simulink model "Logical_Ventilation"  (R2025b)
settings: Solver=VariableStepAuto  StartTime=0.0  StopTime=inf  RelTol=1e-3
PostLoadFcn:
  | load rel_humidity.mat;
  | load rel_humidity_heatedwire.mat;
  | load rel_humidityInput.mat;
libraries: slident x2, SignalEditorBlockLib x1
(part 3 of 3)

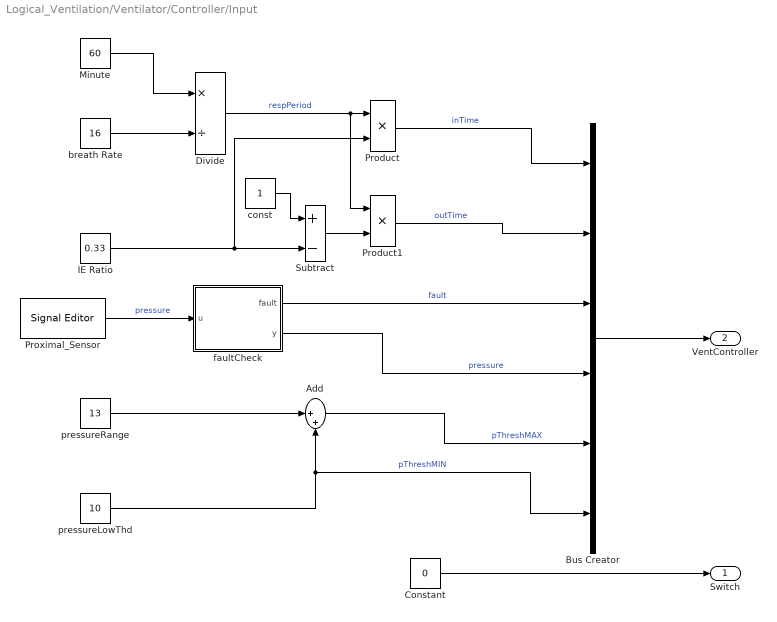
== system Logical_Ventilation/Ventilator/Controller/Input ==
  Add : Sum  Inputs=|++
  Bus Creator : BusCreator  Inputs=6
  Constant : Constant  Value=0
  Divide : Product  Inputs=*/
  IE Ratio : Constant  Value=0.33
  Minute : Constant  Value=60
  Product : Product
  Product1 : Product
  Proximal_Sensor : SignalEditorBlockLib/Signal Editor  FileName=pressure.mat  ActiveScenario=Scenario  ActiveSignal=Signal 1  IsBus=off  OutputBusObjectStr=Bus: BusObject  SampleTime=0  Interpolate=off  ZeroCross=off  OutputAfterFinalValue=Setting to zero  Unit=inherit  PreserveSignalName=on  ApplySigPropsToAllScenarios=on  ApplySigPropsToAllSignals=off  SignalPropertySource=Dialog parameters
  Subtract : Sum  Inputs=+-
  breath Rate : Constant  Value=16
  const : Constant
  faultCheck : MATLAB Function  TreatAsAtomicUnit=on
  pressureLowThd : Constant  Value=10
  pressureRange : Constant  Value=13
  Switch : Outport
  VentController : Outport  Port=2  OutDataTypeStr=Bus: VentController
  wires:
  pressureLowThd/1 -> Add/2, Bus Creator/6  "pThreshMIN"
  faultCheck/2(y) -> Bus Creator/4  "pressure"
  Product/1 -> Bus Creator/1  "inTime"
  faultCheck/1(fault) -> Bus Creator/3  "fault"
  IE Ratio/1 -> Subtract/2, Product/2
  Subtract/1 -> Product1/2
  Proximal_Sensor/1 -> faultCheck/1(u)  "pressure"
  Constant/1 -> Switch/1
  breath Rate/1 -> Divide/2
  const/1 -> Subtract/1
  pressureRange/1 -> Add/1
  Minute/1 -> Divide/1
  Add/1 -> Bus Creator/5  "pThreshMAX"
  Product1/1 -> Bus Creator/2  "outTime"
  Divide/1 -> Product1/1, Product/1  "respPeriod"
  Bus Creator/1 -> VentController/1

== system Logical_Ventilation/Ventilator/Expiratory_System/Expiratory_Tube ==
  Bus Element In1 : Inport  PortName=ExpirTube_Temp
  CheckValve : Subsystem
      settings: PortSchema="{\"entries\":[{\"content\":{\"headerSize\":26,\"margin\":15,\"minimumSpacing\":25,\"sides\":[{\"content\":{},\"type\":\"ConnectorPlacement.EquallySpacedRectSide\",\"uuid\":\"30d5a539-2c7a-40a6-b159-872080309fb0\"},{\"content\":{\"side\":\"RIGHT\"},\"type\":\"ConnectorPlacement.EquallySpacedRectSide\",\"uuid\":\"9c23b845-c6d3-461f-9717-3c81fce4740e\"},{\"content\":{\"side\":\"TOP\"},\"type\":\"ConnectorPlacement.EquallySpacedRectSide\",\"uuid\":\"23e2f61e-2083-47d3-9d3a-aca5cd4f1fc6\"}]},\"type\":\"ConnectorPlacement.EquallySpacedConnector\",\"uuid\":\"a2e9d942-417e-49d1-8834-66036fdf29fe\"}],\"packageUris\":[\"http://schema.mathworks.com/mf0/Connector/R2020b\"],\"version\":\"1.0\"}"
  Temp_RH_Sensor : Subsystem
      settings: PortSchema="{\"entries\":[{\"content\":{\"headerSize\":26,\"margin\":15,\"minimumSpacing\":25,\"sides\":[{\"content\":{},\"type\":\"ConnectorPlacement.EquallySpacedRectSide\",\"uuid\":\"30d5a539-2c7a-40a6-b159-872080309fb0\"},{\"content\":{\"connectorIds\":[\"In1\"],\"side\":\"RIGHT\"},\"type\":\"ConnectorPlacement.EquallySpacedRectSide\",\"uuid\":\"9c23b845-c6d3-461f-9717-3c81fce4740e\"},{\"content\":{\"side\":\"TOP\"},\"type\":\"ConnectorPlacement.EquallySpacedRectSide\",\"uuid\":\"23e2f61e-2083-47d3-9d3a-aca5cd4f1fc6\"}]},\"type\":\"ConnectorPlacement.EquallySpacedConnector\",\"uuid\":\"a2e9d942-417e-49d1-8834-66036fdf29fe\"}],\"packageUris\":[\"http://schema.mathworks.com/mf0/Connector/R2020b\"],\"version\":\"1.0\"}"
  wires:
  Bus Element In1/1 -> Temp_RH_Sensor/1(ExpSens_T)

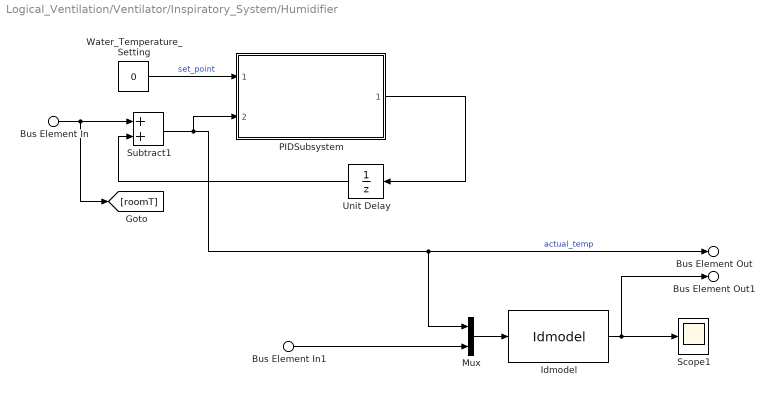
== system Logical_Ventilation/Ventilator/Inspiratory_System/Humidifier ==
  Bus Element In : Inport  PortName=InValveT  Element=Room_T
  Bus Element In1 : Inport  Port=2  PortName=InValveH  Element=Room_H
  Idmodel : slident/Models/Idmodel  sys=mp  IC=0  noi=on  seed=[]
  Mux : Mux  Inputs=2
  PIDSubsystem : Subsystem  ClipboardFcn=|  SystemSampleTime=0.05  ReferencedSubsystem=PIDSubsystem
      | Ts = 0.05;
      | Kp = 0.1;
      | Ki = 0.5;
      settings: PermitHierarchicalResolution=None
  Scope1 : Scope
      settings: ActiveDisplayYMinimum=-0.00289  ActiveDisplayYMaximum=0.02607
  Subtract1 : Sum
  Unit Delay : UnitDelay  SampleTime=-1  HasFrameUpgradeWarning=on
  Water_Temperature_Setting : Constant  Value=0
  Bus Element Out : Outport  PortName=HumidT  Element=Water_T
  Bus Element Out1 : Outport  Port=2  PortName=HumidH  Element=Humidifier_H
  wires:
  PIDSubsystem/1 -> Unit Delay/1
  Unit Delay/1 -> Subtract1/2
  Water_Temperature_Setting/1 -> PIDSubsystem/1  "set_point"
  Bus Element In/1 -> [roomT], Subtract1/1
  Subtract1/1 -> Bus Element Out/1, Mux/1, PIDSubsystem/2  "actual_temp"
  Bus Element In1/1 -> Mux/2
  Idmodel/1 -> Bus Element Out1/1, Scope1/1
  Mux/1 -> Idmodel/1

== system Logical_Ventilation/Ventilator/Inspiratory_System/Inhalation_Valve ==
  Room Relative Humidity (g) : FromWorkspace  VariableName=relh_input  OutDataTypeStr=double
  Room Temp (degC) : Constant  Value=20
  Bus Element Out : Outport  PortName=InspT  Element=Room_T
  Bus Element Out1 : Outport  Port=2  PortName=InspH  Element=Room_H
  wires:
  Room Temp (degC)/1 -> Bus Element Out/1
  Room Relative Humidity (g)/1 -> Bus Element Out1/1

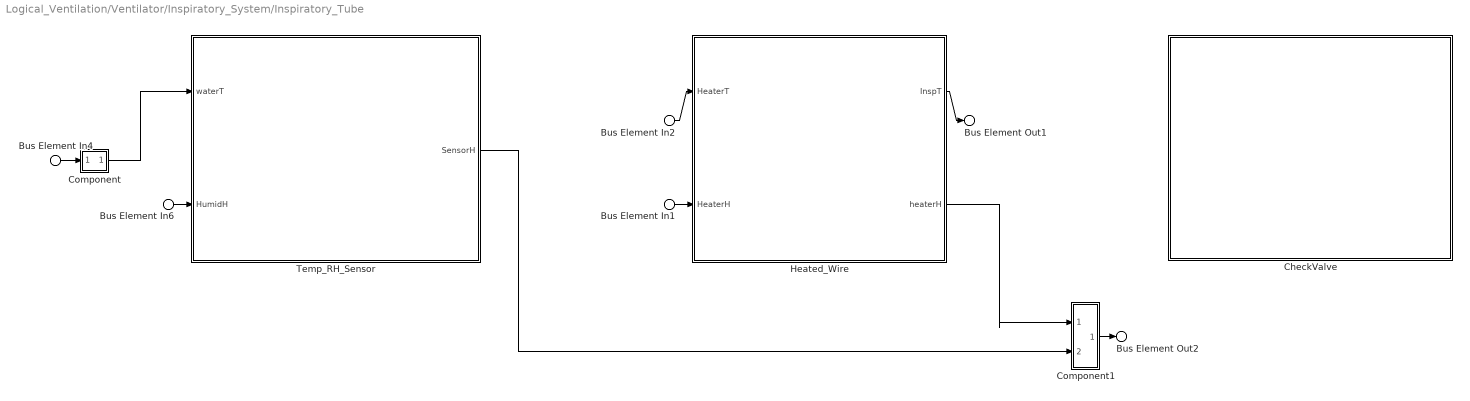
== system Logical_Ventilation/Ventilator/Inspiratory_System/Inspiratory_Tube ==
  Bus Element In1 : Inport  PortName=HumidH
  Bus Element In6 : Inport  PortName=HumidH
  Bus Element In2 : Inport  Port=2  PortName=HumidT
  Bus Element In4 : Inport  Port=2  PortName=HumidT
  CheckValve : Subsystem
      settings: PortSchema="{\"entries\":[{\"content\":{\"headerSize\":26,\"margin\":15,\"minimumSpacing\":25,\"sides\":[{\"content\":{},\"type\":\"ConnectorPlacement.EquallySpacedRectSide\",\"uuid\":\"c28154e5-eaf5-480f-8066-17b2d40a2bdd\"},{\"content\":{\"side\":\"RIGHT\"},\"type\":\"ConnectorPlacement.EquallySpacedRectSide\",\"uuid\":\"c3e70359-248e-4787-971d-b6b9bea98e42\"},{\"content\":{\"side\":\"TOP\"},\"type\":\"ConnectorPlacement.EquallySpacedRectSide\",\"uuid\":\"d2a5be48-e58c-43bd-a458-b63b8b525dc1\"}]},\"type\":\"ConnectorPlacement.EquallySpacedConnector\",\"uuid\":\"4afb880b-0c9a-4048-831b-5d1f8f54d79c\"}],\"packageUris\":[\"http://schema.mathworks.com/mf0/Connector/R2020b\"],\"version\":\"1.0\"}"
  Component : Subsystem
      settings: PortSchema="{\"entries\":[{\"content\":{\"margin\":10,\"minimumSpacing\":15,\"sides\":[{\"content\":{\"connectorIds\":[\"In1\"]},\"type\":\"ConnectorPlacement.EquallySpacedRectSide\",\"uuid\":\"ad8c2344-4809-4832-ae62-0542e39a6856\"},{\"content\":{\"connectorIds\":[\"Out1\"],\"side\":\"RIGHT\"},\"type\":\"ConnectorPlacement.EquallySpacedRectSide\",\"uuid\":\"33082802-14bb-48ab-8efd-54a486fc0ece\"},{\"content\":{\"side\":\"TOP\"},\"type\":\"ConnectorPlacement.EquallySpacedRectSide\",\"uuid\":\"4e03c195-d332-43d0-aeb9-c5e6eda740ab\"}]},\"type\":\"ConnectorPlacement.EquallySpacedConnector\",\"uuid\":\"d0446147-b41e-4bb8-8f56-ac2a90a5b24d\"}],\"packageUris\":[\"http://schema.mathworks.com/mf0/Connector/R2020b\"],\"version\":\"1.0\"}"
  Component1 : Subsystem
      settings: PortSchema="{\"entries\":[{\"content\":{\"margin\":10,\"minimumSpacing\":15,\"sides\":[{\"content\":{\"connectorIds\":[\"In1\",\"In2\"]},\"type\":\"ConnectorPlacement.EquallySpacedRectSide\",\"uuid\":\"18e365e9-4ccc-4943-ae85-7abdeaed82a1\"},{\"content\":{\"connectorIds\":[\"Out1\"],\"side\":\"RIGHT\"},\"type\":\"ConnectorPlacement.EquallySpacedRectSide\",\"uuid\":\"aafe069d-304d-4de7-a3f2-52986cc58723\"},{\"content\":{\"side\":\"TOP\"},\"type\":\"ConnectorPlacement.EquallySpacedRectSide\",\"uuid\":\"efebfcde-c43f-4485-9584-5cc34f249b53\"}]},\"type\":\"ConnectorPlacement.EquallySpacedConnector\",\"uuid\":\"82b97aa5-a7bf-41ea-90eb-26c45b3d9e14\"}],\"packageUris\":[\"http://schema.mathworks.com/mf0/Connector/R2020b\"],\"version\":\"1.0\"}"
  Heated_Wire : Subsystem
      settings: PortSchema="{\"entries\":[{\"content\":{\"headerSize\":26,\"margin\":15,\"minimumSpacing\":25,\"sides\":[{\"content\":{\"connectorIds\":[\"In1\",\"In2\"]},\"type\":\"ConnectorPlacement.EquallySpacedRectSide\",\"uuid\":\"c28154e5-eaf5-480f-8066-17b2d40a2bdd\"},{\"content\":{\"connectorIds\":[\"Out1\",\"Out2\"],\"side\":\"RIGHT\"},\"type\":\"ConnectorPlacement.EquallySpacedRectSide\",\"uuid\":\"c3e70359-248e-4787-971d-b6b9bea98e42\"},{\"content\":{\"side\":\"TOP\"},\"type\":\"ConnectorPlacement.EquallySpacedRectSide\",\"uuid\":\"d2a5be48-e58c-43bd-a458-b63b8b525dc1\"}]},\"type\":\"ConnectorPlacement.EquallySpacedConnector\",\"uuid\":\"4afb880b-0c9a-4048-831b-5d1f8f54d79c\"}],\"packageUris\":[\"http://schema.mathworks.com/mf0/Connector/R2020b\"],\"version\":\"1.0\"}"
  Temp_RH_Sensor : Subsystem
      settings: PortSchema="{\"entries\":[{\"content\":{\"headerSize\":26,\"margin\":15,\"minimumSpacing\":25,\"sides\":[{\"content\":{\"connectorIds\":[\"In1\",\"In2\"]},\"type\":\"ConnectorPlacement.EquallySpacedRectSide\",\"uuid\":\"30d5a539-2c7a-40a6-b159-872080309fb0\"},{\"content\":{\"connectorIds\":[\"Out1\"],\"side\":\"RIGHT\"},\"type\":\"ConnectorPlacement.EquallySpacedRectSide\",\"uuid\":\"9c23b845-c6d3-461f-9717-3c81fce4740e\"},{\"content\":{\"side\":\"TOP\"},\"type\":\"ConnectorPlacement.EquallySpacedRectSide\",\"uuid\":\"23e2f61e-2083-47d3-9d3a-aca5cd4f1fc6\"}]},\"type\":\"ConnectorPlacement.EquallySpacedConnector\",\"uuid\":\"a2e9d942-417e-49d1-8834-66036fdf29fe\"}],\"packageUris\":[\"http://schema.mathworks.com/mf0/Connector/R2020b\"],\"version\":\"1.0\"}"
  Bus Element Out1 : Outport  PortName=InspT
  Bus Element Out2 : Outport  Port=2  PortName=heaterH
  wires:
  Bus Element In2/1 -> Heated_Wire/1(HeaterT)
  Bus Element In1/1 -> Heated_Wire/2(HeaterH)
  Heated_Wire/1(InspT) -> Bus Element Out1/1
  Bus Element In4/1 -> Component/1(HumidT)
  Component/1(waterT) -> Temp_RH_Sensor/1(waterT)
  Heated_Wire/2(heaterH) -> Component1/1(heaterH)
  Bus Element In6/1 -> Temp_RH_Sensor/2(HumidH)
  Temp_RH_Sensor/1(SensorH) -> Component1/2(SensorH)
  Component1/1(Out) -> Bus Element Out2/1

== system Logical_Ventilation/Ventilator/Expiratory_System/Expiratory_Tube/CheckValve ==

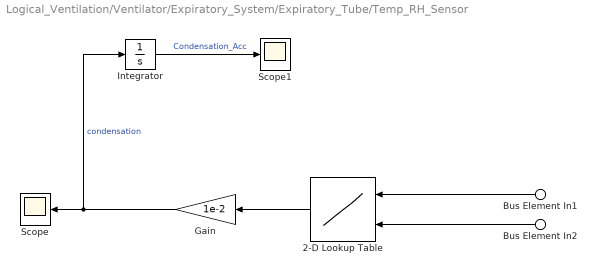
== system Logical_Ventilation/Ventilator/Expiratory_System/Expiratory_Tube/Temp_RH_Sensor ==
  Bus Element In1 : Inport  PortName=ExpSens_T  Element=Water_T
  Bus Element In2 : Inport  PortName=ExpSens_T  Element=heatedWire_T
  2-D Lookup Table : Lookup_n-D  BreakpointsForDimension1=[20 40 45]  BreakpointsForDimension2=[30;37]  Table=[1.75 2.5;2.2 3.1;2.5 3.5]  InternalRulePriority=Speed  RndMeth=Simplest
      settings: InputPortMap=u0,u1
  Gain : Gain  Gain=1e-2
  Integrator : Integrator
  Scope : Scope
      settings: ActiveDisplayYMinimum=-0.0231  ActiveDisplayYMaximum=0.04221
  Scope1 : Scope
      settings: ActiveDisplayYMinimum=-0.20635  ActiveDisplayYMaximum=1.85719
  wires:
  2-D Lookup Table/1 -> Gain/1
  Gain/1 -> Integrator/1, Scope/1  "condensation"
  Bus Element In1/1 -> 2-D Lookup Table/1
  Bus Element In2/1 -> 2-D Lookup Table/2
  Integrator/1 -> Scope1/1  "Condensation_Acc"

== system Logical_Ventilation/Ventilator/Inspiratory_System/Inspiratory_Tube/CheckValve ==

== system Logical_Ventilation/Ventilator/Inspiratory_System/Inspiratory_Tube/Component ==
  In Bus Element : Inport  PortName=HumidT  Element=Water_T
  Out Bus Element : Outport  PortName=waterT  Element=Water_T
  wires:
  In Bus Element/1 -> Out Bus Element/1

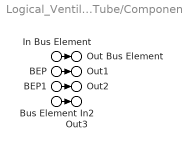
== system Logical_Ventilation/Ventilator/Inspiratory_System/Inspiratory_Tube/Component1 ==
  In Bus Element : Inport  PortName=heaterH  Element=Room_H
  BEP : Inport  PortName=heaterH  Element=Humidifier_H
  BEP1 : Inport  PortName=heaterH  Element=CondLvl
  Bus Element In2 : Inport  Port=2  PortName=SensorH  Element=Insp_Humidity
  Out Bus Element : Outport  PortName=Out  Element=Room_H
  Out1 : Outport  PortName=Out  Element=Humidifier_H
  Out2 : Outport  PortName=Out  Element=CondLvl
  Out3 : Outport  PortName=Out  Element=Insp_Humidity
  wires:
  In Bus Element/1 -> Out Bus Element/1
  BEP/1 -> Out1/1
  BEP1/1 -> Out2/1
  Bus Element In2/1 -> Out3/1

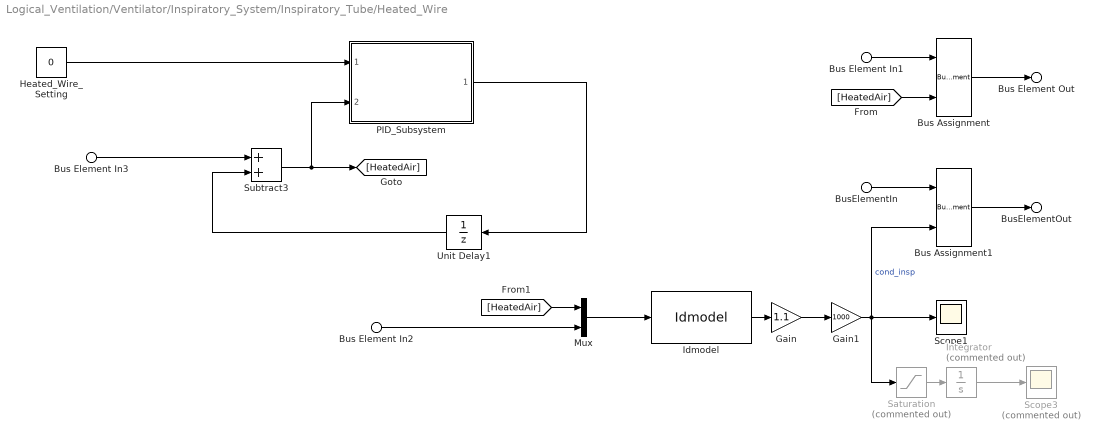
== system Logical_Ventilation/Ventilator/Inspiratory_System/Inspiratory_Tube/Heated_Wire ==
  Bus Element In1 : Inport  PortName=HeaterT
  Bus Element In3 : Inport  PortName=HeaterT  Element=Water_T
  BusElementIn : Inport  Port=2  PortName=HeaterH
  Bus Element In2 : Inport  Port=2  PortName=HeaterH  Element=Humidifier_H
  Bus Assignment : BusAssignment  AssignedSignals=heatedWire_T
  Bus Assignment1 : BusAssignment  AssignedSignals=CondLvl
  Gain : Gain  Gain=1.1
  Gain1 : Gain  Gain=1000
  Heated_Wire_Setting : Constant  Value=0
  Idmodel : slident/Models/Idmodel  sys=mp_heatedwire  IC=0  noi=on  seed=[]
  Integrator : Integrator  Commented=on
  Mux : Mux  Inputs=2
  PID_Subsystem : Subsystem  ReferencedSubsystem=PIDSubsystem
      settings: PermitHierarchicalResolution=None
  Saturation : Saturate  Commented=on  UpperLimit=inf  LowerLimit=0
  Scope1 : Scope
      settings: ActiveDisplayYMinimum=-16.14251  ActiveDisplayYMaximum=26.58007  DataLoggingVariableName=ScopeData3
  Scope3 : Scope  Commented=on
      settings: ActiveDisplayYMinimum=-0.17411  ActiveDisplayYMaximum=1.56698
  Subtract3 : Sum
  Unit Delay1 : UnitDelay  SampleTime=-1  HasFrameUpgradeWarning=on
  Bus Element Out : Outport  PortName=InspT
  BusElementOut : Outport  Port=2  PortName=heaterH
  wires:
  Bus Element In3/1 -> Subtract3/1
  Unit Delay1/1 -> Subtract3/2
  Subtract3/1 -> PID_Subsystem/2, [HeatedAir]
  Mux/1 -> Idmodel/1
  Idmodel/1 -> Gain/1
  Gain/1 -> Gain1/1
  Bus Element In2/1 -> Mux/2
  Bus Element In1/1 -> Bus Assignment/1
  Bus Assignment/1 -> Bus Element Out/1
  [HeatedAir] -> Bus Assignment/2
  [HeatedAir] -> Mux/1
  PID_Subsystem/1 -> Unit Delay1/1
  Integrator/1 -> Scope3/1
  Saturation/1 -> Integrator/1
  Gain1/1 -> Bus Assignment1/2, Saturation/1, Scope1/1  "cond_insp"
  BusElementIn/1 -> Bus Assignment1/1
  Bus Assignment1/1 -> BusElementOut/1
  Heated_Wire_Setting/1 -> PID_Subsystem/1

== system Logical_Ventilation/Ventilator/Inspiratory_System/Inspiratory_Tube/Temp_RH_Sensor ==
  Bus Element In1 : Inport  PortName=waterT
  Bus Element In2 : Inport  Port=2  PortName=HumidH
  1-D Lookup Table : Lookup_n-D  NumberOfTableDimensions=1  BreakpointsForDimension1=[20 25 30 35 40 45]  Table=[0.25 0.3 0.375 0.475 0.6 0.7]  InternalRulePriority=Speed  RndMeth=Simplest
  Bus Assignment : BusAssignment  AssignedSignals=Insp_Humidity
  Gain : Gain  Gain=100
  Bus Element Out : Outport  PortName=SensorH
  wires:
  1-D Lookup Table/1 -> Gain/1
  Bus Element In1/1 -> 1-D Lookup Table/1
  Gain/1 -> Bus Assignment/2  "Inspiration_Humidity"
  Bus Element In2/1 -> Bus Assignment/1
  Bus Assignment/1 -> Bus Element Out/1

== matlab function Logical_Ventilation/Ventilator/Controller/Input/faultCheck ==
  data: fault output; u input; y output
function [fault,y] = FaultCheck(u)
if u < 5 || u > 50
    fault = true;
    y = 25;
else
    fault = false;
    y = u;
end

== stateflow chart Logical_Ventilation/Ventilator/Controller/SupervisoryLogic ==
  state Init
    en: exhaleValve = 0;
    inhaleValve=inhaleValveMax;
    inhaleValveMin=0.0;
    VentFlag = true;
  state OFF
    en:
    VentFlag =false;
  note: Initialise inputs and allow to settle
  state Pressure_InRange
    en:
    PressInRange = true;
    state IN
      en: inhaleValve = inhaleValveMax;
      exhaleValve = 0;
      count = VentController.inTime;
      state PUMP
      state ADJUST
        en: inhaleValve=max(0.0,inhaleValve-deltaFrac);
      (default) -> PUMP
      ADJUST -> PUMP
      PUMP -> ADJUST : [(VentController.pressure > VentController.press_MAX) && (inhaleValve>inhaleValveMin)]
    state OUT
      state VENT
        en: count = VentController.outTime;
        inhaleValve = 0;
        inhaleValveMin=max(0.0,inhaleValveMin-deltaDriftClosed);
        exhaleValve = 1;
      state MAINTAIN_PEEP
        en: exhaleValve = 0;
        inhaleValveMin=inhaleValveMin+deltaFrac;
      (default) -> VENT
      VENT -> MAINTAIN_PEEP : [VentController.pressure < VentController.press_MIN]
    (default) -> IN
    OUT -> IN : [after(count,sec)]
    IN -> OUT : [after(count,sec)]
  note: Must also maintain a minimum pressure
  (default) -> OFF
  Init -> OFF [order 2] : [sw ==0]
  OFF -> Init : [sw ==1]
  Init -> Pressure_InRange [order 1] : [after(1,sec)]
  Pressure_InRange -> Init : [sw == 0]
  data: sw input; VentController input Bus: VentController; deltaFrac local =0.05; deltaDriftClosed local =0.1; inhaleValveMin local; inhaleValveMax local =0.4; count local; PressInRange output boolean; exhaleValve output; inhaleValve output; VentFlag output
